simulink model "power_ResonantLLCConverter_FLi"  (R2020b)
settings: Solver=VariableStepAuto  StartTime=0.0  StopTime=0.03  MaxStep=1e-4  RelTol=1e-4  EnableMultiTasking=on
PreLoadFcn:
  | Rs_fet=1e8;  % FET snubber resistance (ohms)
  | Cs_fet=inf;  % FET snubber capacitance (ohms)
  | Vf=0.6;        % Diode forward voltage (V)
values from neighbouring files (symbols this model uses):
  fr = 1/(2*pi*sqrt(Lr*Cr))    [LLC_converter_design_script.m]    (also in simulation_script.m)
  fs_min = 50e3    (= 50000)    [LLC_converter_design_script.m]    (also in simulation_script.m = 30000)
  Lm = (m-1)*Lr    [LLC_converter_design_script.m]    (also in simulation_script.m = 8.82550835328e-05)
  Lr = 1/((2*pi*fr)^2*Cr)    [LLC_converter_design_script.m]    (also in simulation_script.m = 1.47091805888e-05)
  Po = 10e3    (= 10000)    [LLC_converter_design_script.m]    (also in simulation_script.m)
  ratio_NpNs = 14    [LLC_converter_design_script.m]    (also in simulation_script.m)
  Vin = Vo_pfc    (= 750)    [LLC_converter_design_script.m]    (also in simulation_script.m)
  Vin_min = sqrt(Vo_pfc^2-(2*Pin*Time_hu/C_pfc))    [LLC_converter_design_script.m]    (also in simulation_script.m)
  Vout = 55    [LLC_converter_design_script.m]    (also in simulation_script.m)
undefined symbols (not defined in the file or in its folder): DiscIntNeverNeededParam
libraries: powerlib x29, powerlib_meascontrol x6
Description:
  | Copyright 2008-2019 The MathWorks, Inc.
settings Model: SimulationMode=accelerator  Creator=MathWorks  LastModifiedBy=Temp
settings SolverCC: SolverResetMethod=Robust
settings OptimizationCC: LifeSpan=inf
settings DebuggingCC: ReadBeforeWriteMsg=DisableAll  WriteAfterWriteMsg=DisableAll  WriteAfterReadMsg=DisableAll  MultiTaskDSMMsg=none  SFUnexpectedBacktrackingDiag=warning  SFNoUnconditionalDefaultTransitionDiag=warning  SFExecutionAtInitializationDiag=none  ArithmeticOperatorsInVariantConditions=warning
settings ModelReferenceCC: UpdateModelReferenceTargets=IfOutOfDate
settings SFSimCC: SFSimEcho=off  SimUseLocalCustomCode=off  CustomCodeUndefinedFunction=UseInterfaceOnly
settings RTWCC: RTWUseLocalCustomCode=off
settings CodeAppCC: StateflowObjectComments=on
settings GRTTargetCC: TargetLangStandard=C89/C90 (ANSI)
settings ConfigComp: CovMetricSettings=dw  CovSaveCumulativeToWorkspaceVar=on  CovSaveSingleToWorkspaceVar=on  CovExternalEMLEnable=off
settings SimscapeCC: SimscapeNormalizeSystem=off  SimscapeNominalValues={1, 'bar'; 1, 'cm^3/s'; 1, 'bar*kg/s'; 1, 'kJ/kg'; 1, 'kW'; }

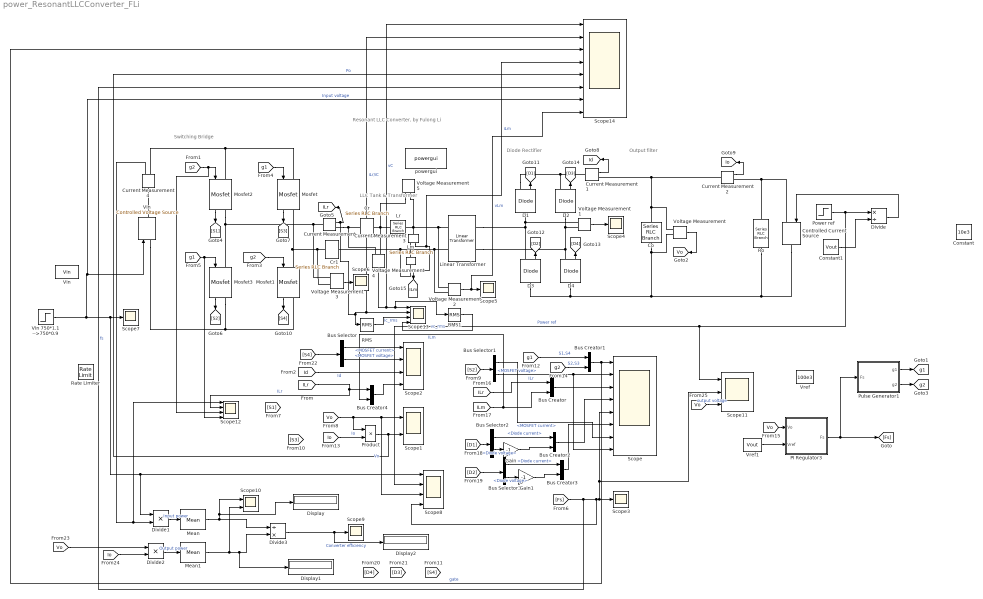
== system power_ResonantLLCConverter_FLi ==
  note: Diode Rectifier
  note: Switching Bridge
  note: Output filter
  note: LLC Tank & Transformer
  note: Resonant LLC Converter, by Fulong Li
  Bus Creator{,1..4} (5 alike) : BusCreator  Inputs=2
  Bus Selector : BusSelector  OutputSignals=MOSFET current,MOSFET voltage
  Bus Selector1 : BusSelector  OutputSignals=MOSFET current,MOSFET voltage
  Bus Selector2 : BusSelector  OutputSignals=Diode current,Diode voltage
  Bus Selector3 : BusSelector  OutputSignals=Diode current,Diode voltage
  Co : powerlib/Elements/Series RLC Branch  LConnTagsString=__new0  RConnTagsString=__new0  BranchType=C  Resistance=1e-4  Inductance=200e-6  SetiL0=off  InitialCurrent=0  Capacitance=470e-6*2  Setx0=on  InitialVoltage=Vout  Measurements=None
  Constant : Constant  Value=10e3
  Constant1 : Constant  Value=Vout
  Controlled Current Source : powerlib/Electrical Sources/Controlled Current Source  Initialize=on  Source_Type=AC  Amplitude=0  Phase=0  Frequency=0  Measurements=None
  Cr : powerlib/Elements/Series RLC Branch  LConnTagsString=__new0  RConnTagsString=__new0  BranchType=C  Resistance=1e-4  Inductance=200e-6  SetiL0=off  InitialCurrent=0  Capacitance=33e-9*4  Setx0=off  InitialVoltage=40  Measurements=None
  Cr1 : powerlib/Elements/Series RLC Branch  LConnTagsString=__new0  RConnTagsString=__new0  BranchType=C  Resistance=1e-4  Inductance=200e-6  SetiL0=off  InitialCurrent=0  Capacitance=33e-9*4  Setx0=off  InitialVoltage=40  Measurements=None
  Current Measurement{,1..4} (5 alike) : powerlib/Measurements/Current Measurement  PhasorSimulation=off  OutputType=Complex  PSBequivalent=0
  D{1..4} (4 alike) : powerlib/Power Electronics/Diode  Ron=Rd_on  Lon=0  Vf=Vf  IC=0  UseSnubber=off  Rs=1e6  Cs=inf  Measurements=on
  Display : Display
  Display1 : Display
  Display2 : Display
  Divide : Product  Inputs=*/
  Divide1 : Product  Inputs=**
  Divide2 : Product  Inputs=**
  Divide3 : Product  Inputs=/*
  Gain : Gain  Gain=-1
  Gain1 : Gain  Gain=-1
  Linear Transformer : powerlib/Elements/Linear Transformer  UNITS=SI  NominalPower=[10e3 fr]  winding1=[1 0 0]  winding2=[1/ratio_NpNs 0 0]  ThreeWindings=off  winding3=[3.15e+05 0.7938 0.084225]  RmLm=[1e4 0]  Measurements=None  DataType=on
  Lm : powerlib/Elements/Series RLC Branch  LConnTagsString=__new0  RConnTagsString=__new0  BranchType=L  Resistance=1e-4  Inductance=Lm  SetiL0=on  InitialCurrent=0  Capacitance=0.94e-6  Setx0=off  InitialVoltage=40  Measurements=Branch current
  Lr : powerlib/Elements/Series RLC Branch  LConnTagsString=__new0  RConnTagsString=__new0  BranchType=L  Resistance=1e-4  Inductance=Lr  SetiL0=off  InitialCurrent=0  Capacitance=0.94e-6  Setx0=off  InitialVoltage=40  Measurements=None
  Mean : powerlib_meascontrol/Measurements/Mean  Freq=1e3  Vinit=0  Ts=1/10000e3
  Mean1 : powerlib_meascontrol/Measurements/Mean  Freq=100e3  Vinit=0  Ts=1/100e3
  Mosfet{,1..3} (4 alike) : powerlib/Power Electronics/Mosfet  Ron=Rds_on  Lon=0  Rd=0  Vfd=mos_vf  IC=0  Rs=1e5  Cs=inf  Measurements=on
  PI Regulator3 : Subsystem
  Power ref : Step  Time=0.01  Before=0.75*Po  After=Po  SampleTime=2.5000e-05
  Product : Product
  Pulse Generator1 : Subsystem
  RMS : powerlib_meascontrol/Measurements/RMS  TrueRMS=on  Freq=1e3  RMSInit=0  Ts=1/10000e3
  RMS1 : powerlib_meascontrol/Measurements/RMS  TrueRMS=on  Freq=1e3  RMSInit=0  Ts=1/10000e3
  Rate Limiter : RateLimiter  RisingSlewLimit=100e3  FallingSlewLimit=-100e3  SampleTimeMode=inherited  InitialCondition=750*1.1
  Ro : powerlib/Elements/Series RLC Branch  LConnTagsString=__new0  RConnTagsString=__new0  BranchType=R  Resistance=100e3  Inductance=200e-6  SetiL0=off  InitialCurrent=0  Capacitance=400e-6  Setx0=off  InitialVoltage=0  Measurements=None
  Scope : Scope  NumInputPorts=8
  Scope1 : Scope  NumInputPorts=2
  Scope10 : Scope  NumInputPorts=2
  Scope11 : Scope  NumInputPorts=3
  Scope{2,8,12..13} (4 alike) : Scope  NumInputPorts=4
  Scope14 : Scope  NumInputPorts=8
  Scope{3..7,9} (6 alike) : Scope
  Vin : Constant  Value=Vin
  Vin 750*1.1 -->750*0.9 : Step  Time=0.02  Before=Vin  After=Vin_min  SampleTime=2.5000e-05
  "Vin " : powerlib/Electrical Sources/Controlled Voltage Source  Initialize=on  Source_Type=DC  Amplitude=0  Phase=0  Frequency=0  Measurements=None
  Voltage Measurement{,1..5} (6 alike) : powerlib/Measurements/Voltage Measurement  PhasorSimulation=off  OutputType=Complex  PSBequivalent=0
  Vref : Constant  Value=100e3
  Vref1 : Constant  Value=Vout
  powergui : powerlib/powergui  Priority=1  SimulationMode=Continuous  SampleTime=50e-6  frequency=60  Iterations=50  frequencyindice=0  Pbase=100e6  ErrMax=1e-4  UnitsV=kV  UnitsW=MW  buscounter=0  FunctionMessages=off  echomessages=off  EnableUseOfTLC=off  CurrentSourceSwitches=off  DisableSnubberDevices=off  DisableRonSwitches=off  DisableVfSwitches=off  DisplayEquations=off  AutomaticDiscreteSolvers=off  SolverType=Tustin/Backward Euler (TBE)  Interpol=off  ExternalGateDelay=off  methode=off  Ts=10  x0status=blocks  SPID=on  SwTol=0  HookPort=off  NonlinearTolerance=0  nMaxIteration=15  ContinueOnMaxIteration=off  RestoreLinks=warning  ResistiveCurrentMeasurement=off  Frange=[0:2:500]  Ylog=off  Xlog=on  ShowGrid=off  save=off  variable=ZData  structure=0  ZoomFFT=off  StartTime=0.0  cycles=1  DisplayStyle=1  fundamental=60  FreqAxis=off  MaxFrequency=1000  frequencyindicesteady=1  RmsSteady=1  display=off
  tag scope: ILm=global, ILr=global, Id=global, Io=global, Vo=global, g1=global, g2=global
  wires:
  [g2] -> Mosfet1/1
  [g1] -> Mosfet/1
  Current Measurement/1 -> RMS/1, Scope13/2, Scope14/2, [ILr]  "iLr/iC"
  Voltage Measurement/1 -> [Vo]
  Current Measurement1/1 -> [Id]
  Current Measurement2/1 -> [Io]
  [Io] -> Product/2  "Io"
  Product/1 -> Scope14/5, Scope1/2  "Po"
  [Vo] -> Product/1, Scope8/3, Scope1/1  "Vo"
  [g2] -> Scope12/3, Mosfet2/1
  [g1] -> Scope12/4, Mosfet3/1
  [ILr] -> Bus Creator4/1, Scope12/2  "ILr"
  [Id] -> Scope2/3  "Id"
  Bus Selector/1 -> Scope2/1  "<MOSFET current>"
  Bus Selector/2 -> Scope2/2  "<MOSFET voltage>"
  Voltage Measurement1/1 -> Scope4/1
  Voltage Measurement3/1 -> Scope6/1
  Voltage Measurement2/1 -> Scope14/8, Scope5/1  "vLm"
  Pulse Generator1/2(g2) -> [g2]
  [Vo] -> PI Regulator3/1(Vo)
  Pulse Generator1/1(g1) -> [g1]
  Constant1/1 -> Divide/2
  Divide/1 -> Controlled Current Source/1
  Mosfet2/1 -> [S1]
  Mosfet3/1 -> [S2]
  Mosfet/1 -> [S3]
  Mosfet1/1 -> [S4]
  D1/1 -> [D1]
  D3/1 -> [D2]
  D2/1 -> [D3]
  D4/1 -> [D4]
  [g1] -> Bus Creator1/1  "S1,S4"
  [g2] -> Bus Creator1/2  "S2,S3"
  [S2] -> Bus Selector1/1
  Bus Selector1/2 -> Scope/8, Scope/2  "<MOSFET voltage>"
  [ILr] -> Bus Creator/1  "ILr"
  Bus Creator/1 -> Scope/3
  Current Measurement3/1 -> Scope14/4, [ILm]  "iLm"
  [ILm] -> Bus Creator4/2, Bus Creator/2  "ILm"
  Bus Creator1/1 -> Scope14/3, Scope/1  "gate"
  Bus Creator2/1 -> Scope/4
  [S4] -> Bus Selector/1
  [D1] -> Bus Selector2/1
  [D2] -> Bus Selector3/1
  Bus Selector2/1 -> Bus Creator2/1  "<Diode current>"
  Vref1/1 -> PI Regulator3/2(Vref)
  Vin 750*1.1 -->750*0.9/1 -> Scope14/7, "Vin "/1, Scope8/1, Divide1/1, Scope7/1  "Input voltage"
  Power ref/1 -> Scope11/1, Scope8/2, Divide/1  "Power ref"
  [Fs] -> Scope14/6, Scope8/4, Scope11/2, Scope/5, Scope3/1  "fs"
  Bus Selector1/1 -> Scope/7  "<MOSFET current>"
  Current Measurement4/1 -> Scope12/1, Divide1/2
  Divide1/1 -> Mean/1  "Input power"
  Divide2/1 -> Mean1/1  "Output power"
  Divide3/1 -> Display2/1, Scope9/1  "Converter efficiency"
  [Vo] -> Divide2/1
  [Io] -> Divide2/2
  [Vo] -> Scope11/3  "output voltage"
  Mean/1 -> Display/1, Scope10/1, Divide3/1
  Mean1/1 -> Scope10/2, Display1/1, Divide3/2
  PI Regulator3/1(Fs) -> Pulse Generator1/1(Fs), [Fs]
  Bus Selector3/2 -> Gain1/1  "<Diode voltage>"
  Bus Creator3/1 -> Scope/6
  Bus Selector3/1 -> Bus Creator3/1  "<Diode current>"
  Bus Selector2/2 -> Gain/1  "<Diode voltage>"
  Gain/1 -> Bus Creator2/2
  Gain1/1 -> Bus Creator3/2
  Bus Creator4/1 -> Scope2/4
  Voltage Measurement4/1 -> RMS1/1, Scope13/1, Scope14/1  "vC"
  RMS/1 -> Scope13/3  "Ic_rms"
  RMS1/1 -> Scope13/4  "vc_rms"
  connections:
  Co/RConn1 -- Voltage Measurement/LConn2 -- Controlled Current Source/RConn1 -- Ro/RConn1 -- D4/LConn1 -- D3/LConn1
  Linear Transformer/RConn1 -- Voltage Measurement1/LConn1 -- D1/LConn1 -- D3/RConn1
  Cr1/RConn1 -- Lm/RConn1 -- Voltage Measurement2/LConn2 -- Linear Transformer/LConn2
  Linear Transformer/RConn2 -- Voltage Measurement1/LConn2 -- D2/LConn1 -- D4/RConn1
  Mosfet2/LConn1 -- Mosfet/LConn1 -- Current Measurement4/RConn1
  "Vin "/LConn1 -- Mosfet3/RConn1 -- Mosfet1/RConn1
  D1/RConn1 -- D2/RConn1 -- Current Measurement1/LConn1
  Voltage Measurement/LConn1 -- Current Measurement2/LConn1 -- Current Measurement1/RConn1 -- Co/LConn1
  Ro/LConn1 -- Controlled Current Source/LConn1 -- Current Measurement2/RConn1
  Voltage Measurement3/LConn1 -- Mosfet2/RConn1 -- Mosfet3/LConn1 -- Current Measurement/LConn1
  Current Measurement/RConn1 -- Cr/LConn1 -- Voltage Measurement4/LConn2
  Linear Transformer/LConn1 -- Voltage Measurement5/LConn2 -- Lr/RConn1 -- Current Measurement3/LConn1 -- Voltage Measurement2/LConn1
  Voltage Measurement4/LConn1 -- Voltage Measurement5/LConn1 -- Lr/LConn1 -- Cr/RConn1
  Current Measurement3/RConn1 -- Lm/LConn1
  "Vin "/RConn1 -- Current Measurement4/LConn1
  Cr1/LConn1 -- Mosfet/RConn1 -- Mosfet1/LConn1 -- Voltage Measurement3/LConn2

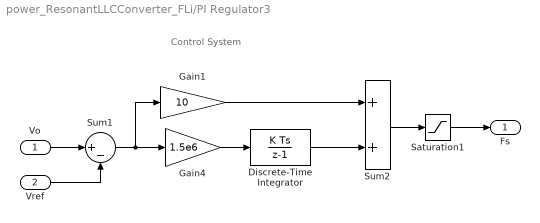
== system power_ResonantLLCConverter_FLi/PI Regulator3 ==
  note: Control System
  Vo : Inport
  Vref : Inport  Port=2
  Discrete-Time Integrator : DiscreteIntegrator  gainval=1  InitialCondition=fr  SampleTime=2.5000e-05  LimitOutput=on  UpperSaturationLimit=300e3  LowerSaturationLimit=fs_min  ICPrevOutput=DiscIntNeverNeededParam  ICPrevScaledInput=DiscIntNeverNeededParam
  Gain1 : Gain  Gain=10  SaturateOnIntegerOverflow=on  OutDataTypeStr=Inherit: Same as input  ParamDataTypeStr=Inherit: Same as input
  Gain4 : Gain  Gain=1.5e6  SaturateOnIntegerOverflow=on  OutDataTypeStr=Inherit: Same as input  ParamDataTypeStr=Inherit: Same as input
  Saturation1 : Saturate  UpperLimit=300e3  LowerLimit=fs_min
  Sum1 : Sum  Inputs=|+-  InputSameDT=on  SaturateOnIntegerOverflow=on  OutDataTypeStr=Inherit: Same as first input
  Sum2 : Sum  InputSameDT=on  SaturateOnIntegerOverflow=on  OutDataTypeStr=Inherit: Same as first input
  Fs : Outport  VectorParamsAs1DForOutWhenUnconnected=off
  wires:
  Saturation1/1 -> Fs/1
  Gain1/1 -> Sum2/1
  Sum2/1 -> Saturation1/1
  Discrete-Time Integrator/1 -> Sum2/2
  Gain4/1 -> Discrete-Time Integrator/1
  Sum1/1 -> Gain4/1, Gain1/1
  Vref/1 -> Sum1/2
  Vo/1 -> Sum1/1

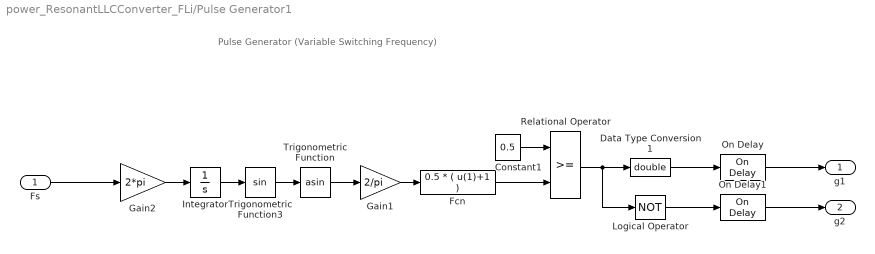
== system power_ResonantLLCConverter_FLi/Pulse Generator1 ==
  note: Pulse Generator
      | (Variable Switching Frequency)
  Fs : Inport
  Constant1 : Constant  Value=0.5
  Data Type Conversion1 : DataTypeConversion  OutDataTypeStr=double
  Fcn : Fcn  Expr=0.5 * ( u(1)+1 )
  Gain1 : Gain  Gain=2/pi  SaturateOnIntegerOverflow=on  OutDataTypeStr=Inherit: Same as input  ParamDataTypeStr=Inherit: Same as input
  Gain2 : Gain  Gain=2*pi  SaturateOnIntegerOverflow=on  OutDataTypeStr=Inherit: Same as input  ParamDataTypeStr=Inherit: Same as input
  Integrator : Integrator
  Logical Operator : Logic  Operator=NOT  AllPortsSameDT=off  OutDataTypeStr=float('double')
  On Delay : powerlib_meascontrol/Logic/On Delay  DelayType=On delay  delay=deadtime  ic=0  Ts=0
  On Delay1 : powerlib_meascontrol/Logic/On Delay  DelayType=On delay  delay=deadtime  ic=0  Ts=0
  Relational Operator : RelationalOperator  OutDataTypeStr=boolean  RndMeth=Nearest
  Trigonometric Function : Trigonometry  Operator=asin
  Trigonometric Function3 : Trigonometry
  g1 : Outport  VectorParamsAs1DForOutWhenUnconnected=off
  g2 : Outport  Port=2  VectorParamsAs1DForOutWhenUnconnected=off
  wires:
  On Delay1/1 -> g2/1
  On Delay/1 -> g1/1
  Fs/1 -> Gain2/1
  Gain2/1 -> Integrator/1
  Data Type Conversion1/1 -> On Delay/1
  Logical Operator/1 -> On Delay1/1
  Fcn/1 -> Relational Operator/2
  Relational Operator/1 -> Logical Operator/1, Data Type Conversion1/1
  Constant1/1 -> Relational Operator/1
  Integrator/1 -> Trigonometric Function3/1
  Trigonometric Function/1 -> Gain1/1
  Gain1/1 -> Fcn/1
  Trigonometric Function3/1 -> Trigonometric Function/1
